simulink subsystem "AxialAccelerationSubsystem"  (R2023b)
settings: Solver=VariableStepAuto  StartTime=0.0  StopTime=10.0  RelTol=1e-3
values from neighbouring files (symbols this model uses):
  m = weight/g    (= 0.815494393476)    [drone_input_params.m]
settings Model: Creator=FRESH  LastModifiedBy=FRESH

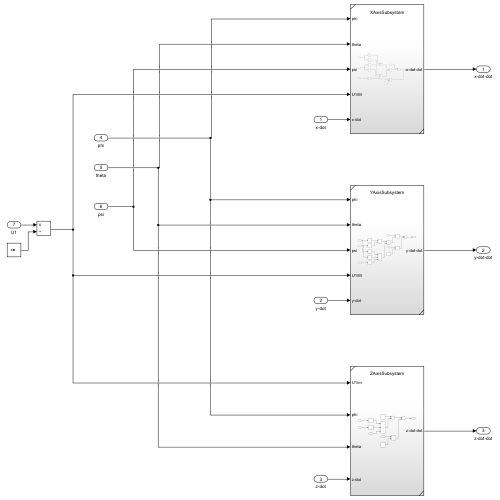
[thumbnail: Simulink's stored preview of the top-level diagram]
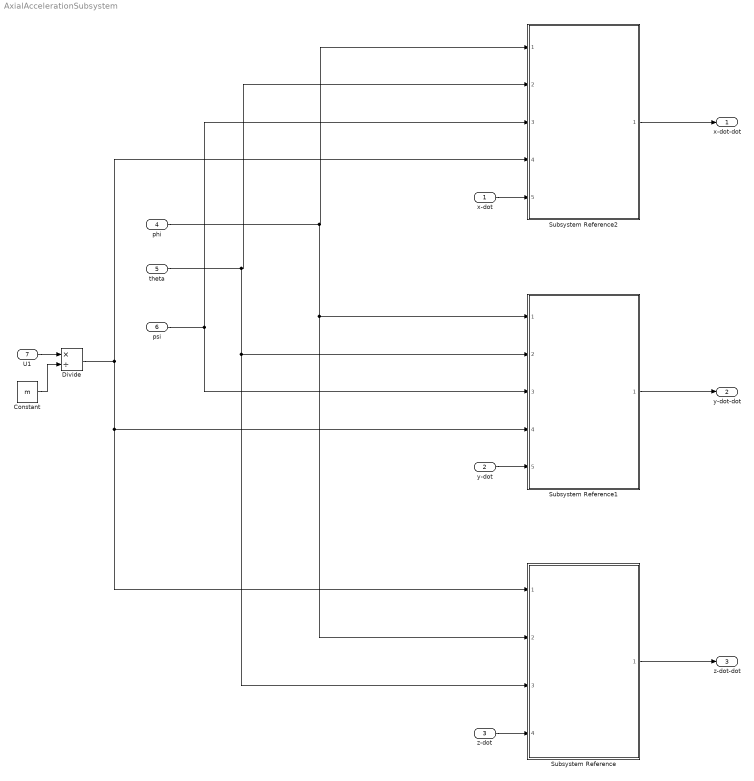
== system AxialAccelerationSubsystem ==
  x-dot : Inport
  y-dot : Inport  Port=2
  z-dot : Inport  Port=3
  phi : Inport  Port=4
  theta : Inport  Port=5
  psi : Inport  Port=6
  U1 : Inport  Port=7
  Constant : Constant  Value=m
  Divide : Product  Inputs=*/
  Subsystem Reference : Subsystem  ReferencedSubsystem=ZAxisSubsystem
  Subsystem Reference1 : Subsystem  ReferencedSubsystem=YAxisSubsystem
  Subsystem Reference2 : Subsystem  ReferencedSubsystem=XAxisSubsystem
  x-dot-dot : Outport
  y-dot-dot : Outport  Port=2
  z-dot-dot : Outport  Port=3
  wires:
  U1/1 -> Divide/1
  Constant/1 -> Divide/2
  x-dot/1 -> Subsystem Reference2/5
  y-dot/1 -> Subsystem Reference1/5
  z-dot/1 -> Subsystem Reference/4
  phi/1 -> Subsystem Reference/2, Subsystem Reference1/1, Subsystem Reference2/1
  theta/1 -> Subsystem Reference/3, Subsystem Reference1/2, Subsystem Reference2/2
  psi/1 -> Subsystem Reference2/3, Subsystem Reference1/3
  Divide/1 -> Subsystem Reference2/4, Subsystem Reference/1, Subsystem Reference1/4
  Subsystem Reference2/1 -> x-dot-dot/1
  Subsystem Reference1/1 -> y-dot-dot/1
  Subsystem Reference/1 -> z-dot-dot/1
